simulink model "PM_fnc10_DevHarness_Power_Limit_2Dlookup"  (R2022a)
settings: Solver=FixedStepAuto  StartTime=0.0  StopTime=10.0  FixedStep=1  RelTol=1e-3
undefined symbols (not defined in the file or in its folder): cal_table01_xtempysoc_cell_dischg_limits_A, cal_table_cell_soc_percent, cal_table_cell_temp_degC
settings Model: Creator=306427  LastModifiedBy=306427
settings OptimizationCC: DefaultParameterBehavior=Inlined  EnhancedBackFolding=on  PassReuseOutputArgsAs=Individual arguments  ZeroExternalMemoryAtStartup=off  ZeroInternalMemoryAtStartup=off  OptimizeBlockOrder=speed  DifferentSizesBufferReuse=on  OptimizationCustomize=off  EfficientTunableParamExpr=on
settings DebuggingCC: ParameterTunabilityLossMsg=error
settings SFSimCC: MATLABDynamicMemAlloc=off
settings RTWCC: SystemTargetFile=ert.tlc  GenCodeOnly=on  TemplateMakefile=ert_default_tmf
settings CodeAppCC: ForceParamTrailComments=on  IgnoreCustomStorageClasses=off  OperatorAnnotations=on  SimulinkDataObjDesc=on  SFDataObjDesc=on  InsertBlockDesc=on
settings ERTTargetCC: TargetLangStandard=C99 (ISO)  GenerateSampleERTMain=on  InlinedParameterPlacement=NonHierarchical  ERTCustomFileTemplate=example_file_process.tlc

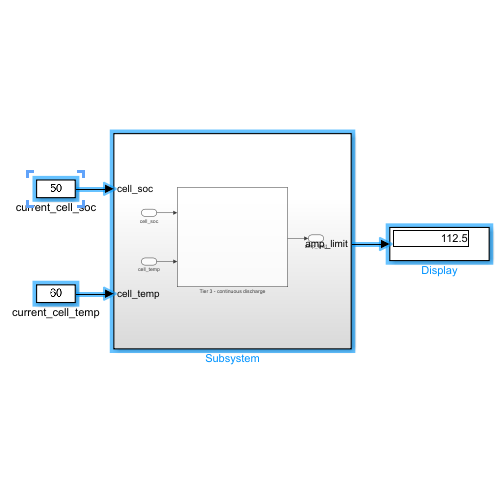
[thumbnail: Simulink's stored preview of the top-level diagram]
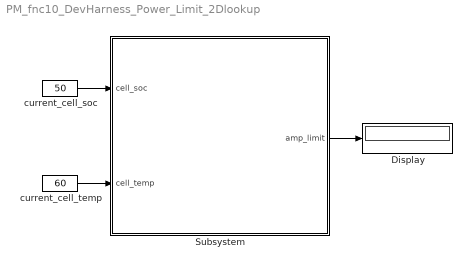
== system PM_fnc10_DevHarness_Power_Limit_2Dlookup ==
  Display : Display
  Subsystem : Subsystem
  current_cell_soc : Constant  Value=50
  current_cell_temp : Constant  Value=60
  wires:
  current_cell_soc/1 -> Subsystem/1(cell_soc)
  current_cell_temp/1 -> Subsystem/2(cell_temp)
  Subsystem/1(amp_limit) -> Display/1

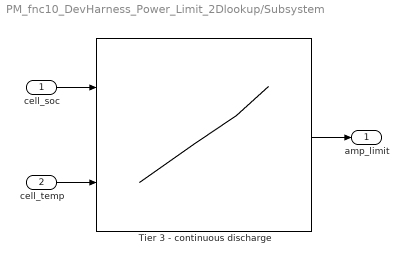
== system PM_fnc10_DevHarness_Power_Limit_2Dlookup/Subsystem ==
  cell_soc : Inport
  cell_temp : Inport  Port=2
  Tier 3 - continuous discharge : Lookup_n-D  BreakpointsForDimension1=cal_table_cell_soc_percent  BreakpointsForDimension2=cal_table_cell_temp_degC  Table=cal_table01_xtempysoc_cell_dischg_limits_A  InternalRulePriority=Speed  RndMeth=Simplest
      settings: InputPortMap=u0,u1
  amp_limit : Outport
  wires:
  cell_soc/1 -> Tier 3 - continuous discharge/1
  Tier 3 - continuous discharge/1 -> amp_limit/1
  cell_temp/1 -> Tier 3 - continuous discharge/2
